simulink model "IP_LQG_MIO16E4_2015a"  (R2025b)
settings: Solver=ode3  StartTime=0.0  StopTime=200  RelTol=1e-3  EnableMultiTasking=on
values from neighbouring files (symbols this model uses):
  ALPHA_MAX = 90 * pi/180    (= 1.57079632679)    [IP_MACRO.m]
  BETA_MAX = 15 * pi/180    (= 0.261799387799)    [IP_MACRO.m]
  K_i = K_aug(6)    [IP_MACRO.m]
  K_x = K_aug(1:5)    [IP_MACRO.m]
  L = lqe(A, G, C, Qe, Re)    [IP_MACRO.m]
  TIME_DELAY = 6    [IP_MACRO.m]
  Ts = 0.001    [IP_MACRO.m]
  V_MAX = 5    [IP_MACRO.m]
  V_MIN = -5    [IP_MACRO.m]
undefined symbols (not defined in the file or in its folder): A, B, C, MIO, National_Instruments, PCI
libraries: sldrtlib x3, simulink x2
settings Model: SimulationMode=external  ExtModeTrigDuration=100000  Creator=Alunos  LastModifiedBy=Asus
settings SolverCC: AlgebraicLoopSolver=TrustRegion
settings DataIOCC: LimitDataPoints=on  SaveFormat=Array  ReturnWorkspaceOutputs=off
settings OptimizationCC: LifeSpan=inf
settings DebuggingCC: UnconnectedInputMsg=warning  UnconnectedOutputMsg=warning  UnconnectedLineMsg=warning  SFUnexpectedBacktrackingDiag=warning  SFNoUnconditionalDefaultTransitionDiag=warning  SFExecutionAtInitializationDiag=none  ArithmeticOperatorsInVariantConditions=warning
settings HardwareCC: ProdBitPerPointer=32.0  ProdBitPerSizeT=32.0  ProdBitPerPtrDiffT=32.0  ProdLargestAtomicFloat=None  ProdWordSize=32.0  ProdHWDeviceType=Intel->x86/Pentium  TargetIntDivRoundTo=Zero  TargetEndianess=LittleEndian  TargetHWDeviceType=Intel->x86/Pentium
settings ModelReferenceCC: PropagateSignalLabelsOutOfModel=off
settings SFSimCC: SimUseLocalCustomCode=off  CustomCodeUndefinedFunction=UseInterfaceOnly
settings RTWCC: SystemTargetFile=rtwin.tlc  TemplateMakefile=rtwin.tmf  RTWUseLocalCustomCode=off  RTWCompilerOptimization=on  GPUComputeCapability=3.5  Description=Simulink Desktop Real-Time
settings CodeAppCC: MaxIdLength=95.0  StateflowObjectComments=on
settings STFCustomTargetCC: SystemTargetFile=rtwin.tlc  TargetLangStandard=C99 (ISO)  ModelReferenceCompliant=off  ConcurrentExecutionCompliant=off  MATLABClassNameForMDSCustomization=Simulink.SoftwareTarget.TargetSpecificTriggerConfigurationBase
settings ConfigComp: CovMetricSettings=dw  CovSaveCumulativeToWorkspaceVar=on  CovSaveSingleToWorkspaceVar=on  CovExternalEMLEnable=off

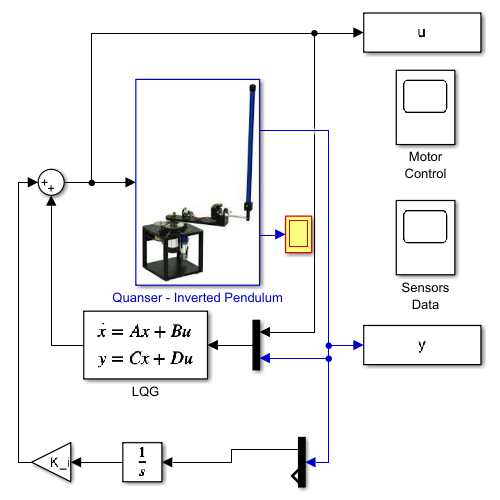
[thumbnail: Simulink's stored preview of the top-level diagram]
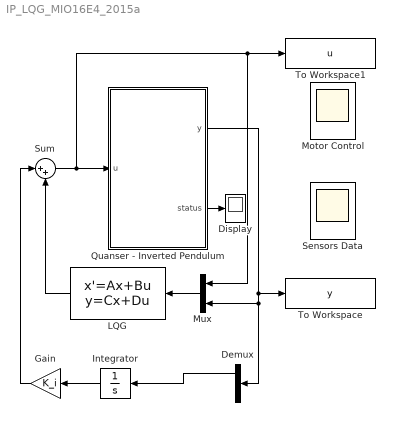
== system IP_LQG_MIO16E4_2015a ==
  Demux : Demux  Outputs=2
  Display : Display
  Gain : Gain  Gain=K_i
  Integrator : Integrator
  LQG : StateSpace  A=A-L*C  B=[B, L]  C=-K_x  D=zeros(1, 1 + size(C, 1))  InitialCondition=0
  Motor Control : Scope
      settings: IsFloating=on  Floating=on  DataLoggingVariableName=ScopeData2
  Mux : Mux  Inputs=2
  Quanser - Inverted Pendulum : Subsystem
      mask Display: image('IP_QUANSER.jpg');
  Sensors Data : Scope
      settings: IsFloating=on  Floating=on  ActiveDisplayYMinimum=-3.1915926535897929  ActiveDisplayYMaximum=3.1915926535897929
  Sum : Sum  Inputs=|++
  To Workspace : ToWorkspace  VariableName=y  SampleTime=-1
  To Workspace1 : ToWorkspace  VariableName=u  SampleTime=-1
  wires:
  Quanser - Inverted Pendulum/1(y) -> Mux/2, Demux/1, To Workspace/1
  LQG/1 -> Sum/2
  Quanser - Inverted Pendulum/2(status) -> Display/1
  Sum/1 -> Mux/1, To Workspace1/1, Quanser - Inverted Pendulum/1(u)
  Demux/1 -> Integrator/1
  Integrator/1 -> Gain/1
  Gain/1 -> Sum/1
  Mux/1 -> LQG/1

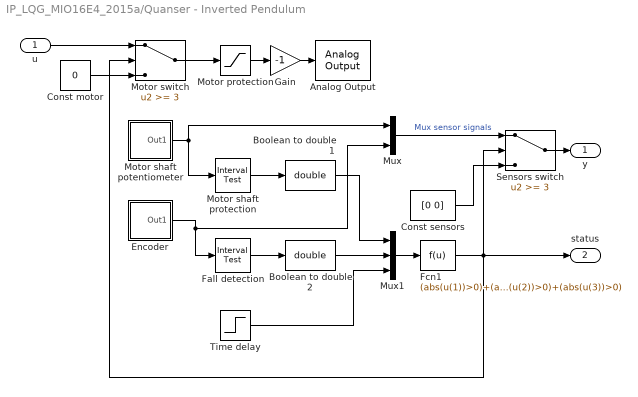
== system IP_LQG_MIO16E4_2015a/Quanser - Inverted Pendulum ==
  u : Inport
  Analog Output : sldrtlib/Analog Output  SampleTime=Ts  MaxMissedTicks=10  ShowMissedTicks=off  YieldWhenWaiting=off  DrvName=National_Instruments/PCI-MIO-16E-4  DrvAddress=4294967295  DrvOptions=[0 0 0 0 0 0]  Channels=1  RangeMode=1  VoltRange=1  InitialValue=0  FinalValue=0
      settings: AttributesFormatString=National Instruments\nPCI-MIO-16E-4 [auto]
  Boolean to double 1 : DataTypeConversion  OutDataTypeStr=double  SaturateOnIntegerOverflow=off  RndMeth=Floor
  Boolean to double 2 : DataTypeConversion  OutDataTypeStr=double  SaturateOnIntegerOverflow=off  RndMeth=Floor
  Const motor : Constant  Value=0
  Const sensors : Constant  Value=[0 0]
  Encoder : Subsystem
  Fall detection : simulink/Logic and Bit Operations/Interval Test  IntervalClosedRight=on  uplimit=BETA_MAX  IntervalClosedLeft=on  lowlimit=-BETA_MAX  OutDataTypeStr=uint8
  Fcn1 : Fcn  Expr=(abs(u(1))>0)+(abs(u(2))>0)+(abs(u(3))>0)
  Gain : Gain  Gain=-1
  Motor protection : Saturate  UpperLimit=V_MAX  LowerLimit=V_MIN
  Motor shaft potentiometer : Subsystem
  Motor shaft protection : simulink/Logic and Bit Operations/Interval Test  IntervalClosedRight=on  uplimit=ALPHA_MAX  IntervalClosedLeft=on  lowlimit=-ALPHA_MAX  OutDataTypeStr=uint8
  Motor switch : Switch  Threshold=3  SaturateOnIntegerOverflow=off  InputSameDT=off
  Mux : Mux  Inputs=2
  Mux1 : Mux  Inputs=3
  Sensors switch : Switch  Threshold=3  SaturateOnIntegerOverflow=off  InputSameDT=off
  Time delay : Step  Time=TIME_DELAY  SampleTime=0
  y : Outport
  status : Outport  Port=2
  wires:
  u/1 -> Motor switch/1
  Motor switch/1 -> Motor protection/1
  Const motor/1 -> Motor switch/3
  Motor shaft potentiometer/1(Out1) -> Mux/1, Motor shaft protection/1
  Encoder/1(Out1) -> Fall detection/1, Mux/2
  Mux1/1 -> Fcn1/1
  Time delay/1 -> Mux1/3
  Fall detection/1 -> Boolean to double 2/1
  Boolean to double 2/1 -> Mux1/2
  Motor shaft protection/1 -> Boolean to double 1/1
  Boolean to double 1/1 -> Mux1/1
  Const sensors/1 -> Sensors switch/3
  Mux/1 -> Sensors switch/1  "Mux sensor signals"
  Sensors switch/1 -> y/1
  Gain/1 -> Analog Output/1
  Motor protection/1 -> Gain/1
  Fcn1/1 -> status/1, Motor switch/2, Sensors switch/2

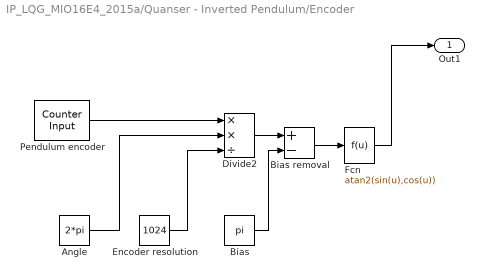
== system IP_LQG_MIO16E4_2015a/Quanser - Inverted Pendulum/Encoder ==
  Angle : Constant  Value=2*pi
  Bias : Constant  Value=pi
  Bias removal : Sum  Inputs=+-
  Divide2 : Product  Inputs=**/
  Encoder resolution : Constant  Value=1024
  Fcn : Fcn  Expr=atan2(sin(u),cos(u))
  Pendulum encoder : sldrtlib/Counter Input  SampleTime=Ts  MaxMissedTicks=10  ShowMissedTicks=off  YieldWhenWaiting=off  DrvName=National_Instruments/PCI-MIO-16E-4  DrvAddress=4294967295  DrvOptions=[0 0 0 0 1 0]  Channels=2  ResetMode=1  CounterEdge=1  CounterGate=1  DataType=1
      settings: AttributesFormatString=National Instruments\nPCI-MIO-16E-4 [auto]
  Out1 : Outport
  wires:
  Bias/1 -> Bias removal/2
  Encoder resolution/1 -> Divide2/3
  Divide2/1 -> Bias removal/1
  Fcn/1 -> Out1/1
  Pendulum encoder/1 -> Divide2/1
  Bias removal/1 -> Fcn/1
  Angle/1 -> Divide2/2

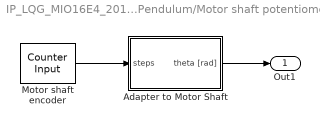
== system IP_LQG_MIO16E4_2015a/Quanser - Inverted Pendulum/Motor shaft potentiometer ==
  Adapter to Motor Shaft : Subsystem
  Motor shaft encoder : sldrtlib/Counter Input  SampleTime=Ts  MaxMissedTicks=10  ShowMissedTicks=off  YieldWhenWaiting=off  DrvName=National_Instruments/PCI-MIO-16E-4  DrvAddress=4294967295  DrvOptions=[0 0 0 0 1 0]  Channels=1  ResetMode=1  CounterEdge=1  CounterGate=1  DataType=1
      settings: AttributesFormatString=National Instruments\nPCI-MIO-16E-4 [auto]
  Out1 : Outport
  wires:
  Motor shaft encoder/1 -> Adapter to Motor Shaft/1(steps)
  Adapter to Motor Shaft/1(theta [rad]) -> Out1/1

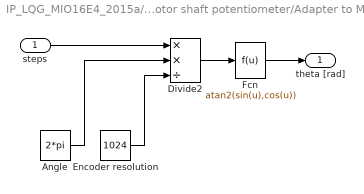
== system IP_LQG_MIO16E4_2015a/Quanser - Inverted Pendulum/Motor shaft potentiometer/Adapter to Motor Shaft ==
  steps : Inport
  Angle : Constant  Value=2*pi
  Divide2 : Product  Inputs=**/
  Encoder resolution : Constant  Value=1024
  Fcn : Fcn  Expr=atan2(sin(u),cos(u))
  theta [rad] : Outport
  wires:
  Angle/1 -> Divide2/2
  Encoder resolution/1 -> Divide2/3
  steps/1 -> Divide2/1
  Divide2/1 -> Fcn/1
  Fcn/1 -> theta [rad]/1
